simulink model "AIV_robot"  (R2024b)
settings: Solver=VariableStepAuto  StartTime=0.0  StopTime=35  RelTol=1e-2
InitFcn:
  | %% Position Error parameter
  | goal_x = 18.5;
  | goal_y = 16;
  | 
  | s0 = sqrt(goal_x^2 + goal_y^2);
  | isGoal_dist = 1.0;
  | 
  | %% Velocity parameter
  | VelScaler = 15;
  | 
  | 
  | %% get bus
  | BusActors = Simulink.Bus;
  | BusActors = getBusActors(BusActors);
  | BusActorsActors = Simulink.Bus;
  | BusActorsActors= getBusActorsActors(BusActorsActors);
  | 
  | %% get agent
  | load("agent.mat")
model workspace (MAT data in the model file):
  firstWarning = 1
  originalScenarioChecksum = '7C1E912B2141DACB6907C14F620C989B'
libraries: simulink x13, drivingscenarioandsensors x8, simulink_extras x1, autolibshared x1, rllib x1
(part 1 of 9)
settings Model: Creator=9  LastModifiedBy=aa007
settings SolverCC: DateTimeAtSimulationTimeZero=[]  ZeroCrossControl=EnableAll  ZeroCrossAlgorithm=Adaptive  MinimalZcImpactIntegration=on
settings DebuggingCC: ParameterOverflowMsg=warning  ParameterPrecisionLossMsg=none

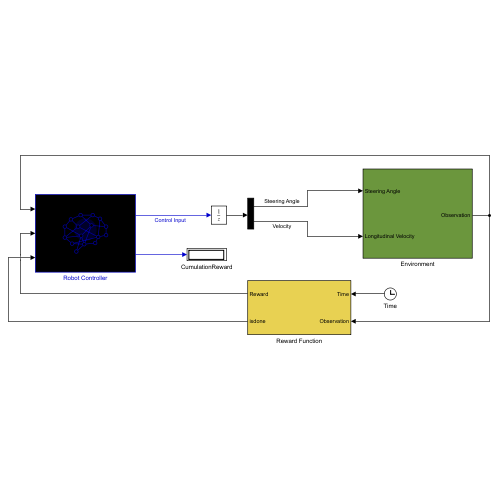
[thumbnail: Simulink's stored preview of the top-level diagram]
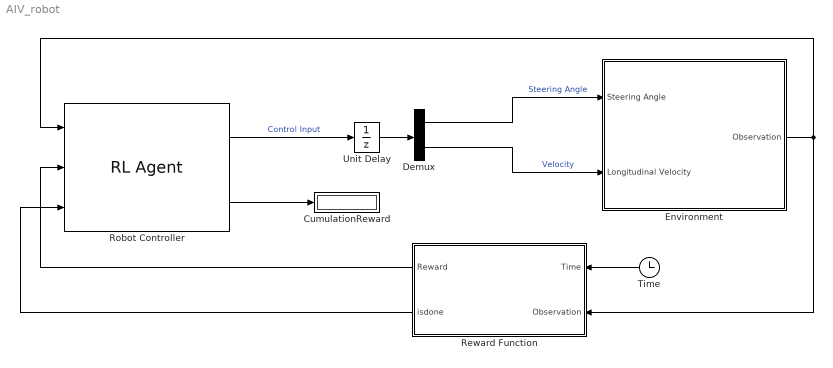
== system AIV_robot ==
  CumulationReward : Display
  Demux : Demux  Outputs=2
  Environment : Subsystem
  Reward Function : Subsystem
  Robot Controller : rllib/RL Agent  Agent=agent  ExternalActionAsInput=off  ProvideLastAction=off  ProvideCumRwd=on  TreatAsDirectFeedthrough=on  UseStrictObservationDataTypes=off
  Time : Clock
  Unit Delay : UnitDelay  SampleTime=-1  HasFrameUpgradeWarning=on
  wires:
  Reward Function/1(Reward) -> Robot Controller/2
  Demux/1 -> Environment/1(Steering Angle)  "Steering Angle"
  Demux/2 -> Environment/2(Longitudinal Velocity)  "Velocity"
  Time/1 -> Reward Function/1(Time)
  Environment/1(Observation) -> Reward Function/2(Observation), Robot Controller/1
  Reward Function/2(isdone) -> Robot Controller/3
  Robot Controller/2 -> CumulationReward/1
  Robot Controller/1 -> Unit Delay/1  "Control Input"
  Unit Delay/1 -> Demux/1

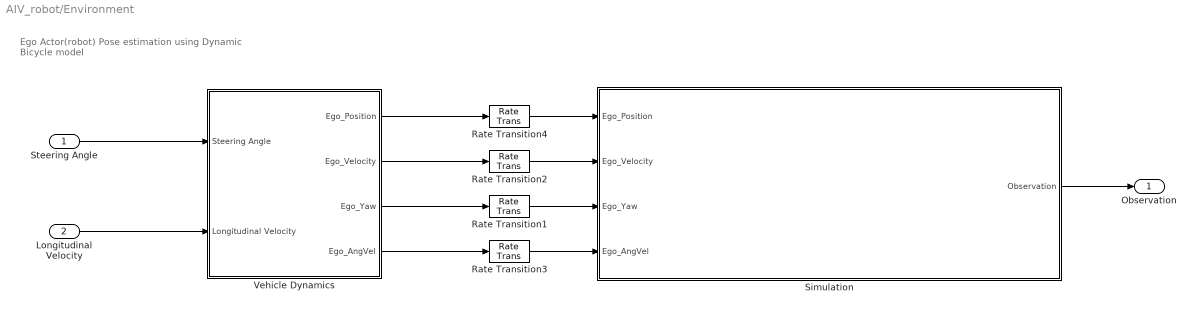
== system AIV_robot/Environment ==
  note: Ego Actor(robot) Pose estimation
      | using Dynamic Bicycle model
  Steering Angle : Inport
  Longitudinal Velocity : Inport  Port=2
  Rate Transition{1..4} (4 alike) : RateTransition
  Simulation : Subsystem
  Vehicle Dynamics : Subsystem
  Observation : Outport
  wires:
  Vehicle Dynamics/1(Ego_Position) -> Rate Transition4/1
  Vehicle Dynamics/2(Ego_Velocity) -> Rate Transition2/1
  Vehicle Dynamics/3(Ego_Yaw) -> Rate Transition1/1
  Vehicle Dynamics/4(Ego_AngVel) -> Rate Transition3/1
  Steering Angle/1 -> Vehicle Dynamics/1(Steering Angle)
  Longitudinal Velocity/1 -> Vehicle Dynamics/2(Longitudinal Velocity)
  Simulation/1(Observation) -> Observation/1
  Rate Transition2/1 -> Simulation/2(Ego_Velocity)
  Rate Transition1/1 -> Simulation/3(Ego_Yaw)
  Rate Transition3/1 -> Simulation/4(Ego_AngVel)
  Rate Transition4/1 -> Simulation/1(Ego_Position)

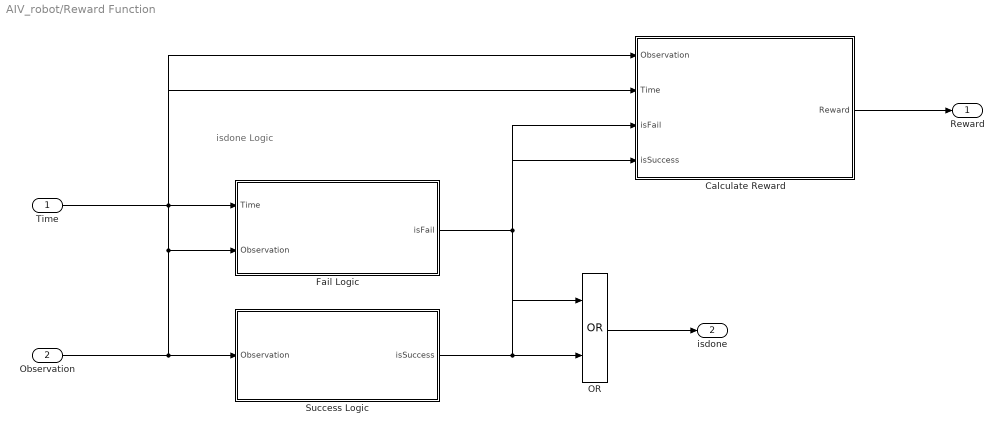
== system AIV_robot/Reward Function ==
  note: isdone Logic
  Time : Inport
  Observation : Inport  Port=2
  Calculate Reward : Subsystem
  Fail Logic : Subsystem
  OR : Logic  Operator=OR  AllPortsSameDT=off  OutDataTypeStr=boolean
  Success Logic : Subsystem
  Reward : Outport
  isdone : Outport  Port=2
  wires:
  Time/1 -> Fail Logic/1(Time), Calculate Reward/2(Time)
  Observation/1 -> Calculate Reward/1(Observation), Fail Logic/2(Observation), Success Logic/1(Observation)
  Fail Logic/1(isFail) -> OR/1, Calculate Reward/3(isFail)
  Success Logic/1(isSuccess) -> Calculate Reward/4(isSuccess), OR/2
  OR/1 -> isdone/1
  Calculate Reward/1(Reward) -> Reward/1

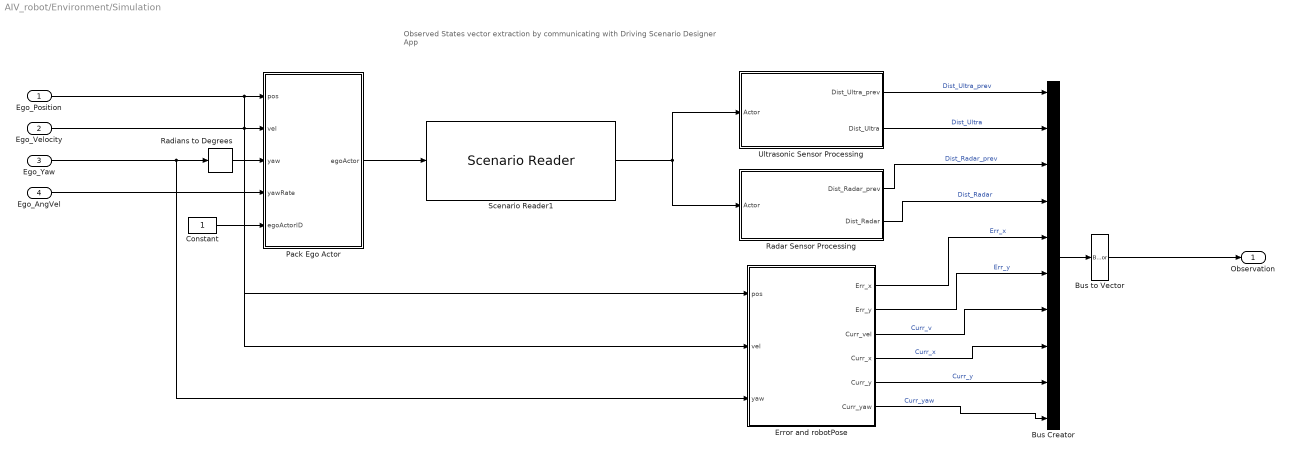
== system AIV_robot/Environment/Simulation ==
  note: Observed States vector extraction
      | by communicating with Driving Scenario Designer App
  Ego_Position : Inport
  Ego_Velocity : Inport  Port=2
  Ego_Yaw : Inport  Port=3
  Ego_AngVel : Inport  Port=4
  Bus Creator : BusCreator  Inputs=10
  Bus to Vector : BusToVector
  Constant : Constant
  Error and robotPose : Subsystem
  Pack Ego Actor : MATLAB Function  Priority=-1  TreatAsAtomicUnit=on
  Radar Sensor Processing : Subsystem
  Radians to Degrees : simulink_extras/Transformations/Radians to Degrees
  Scenario Reader1 : drivingscenarioandsensors/Scenario Reader  Priority=-1  ScenarioSource=From file  ScenarioFileName=C:\Users\aa007\OneDrive\바탕화~1-DESKTOP-L2TT5UE-65992184\ai_ws\ai_ws\scenario.mat  ScenarioVariableName=data  OutputCoordinateSystem=Vehicle coordinates  EgoVehicleSource=Input port  EgoVehicleActorID=1  OrientVehiclesOnRoad=on  OutputEgoVehiclePose=off  OutputEgoVehicleState=off  SampleTime=0.1  LaneBoundaryOutput=None  LaneBoundaryDistance=0:0.5:9.5  LaneBoundaryLocation=Center of lane markings  BusNameSource=Auto  BusName=BusActors  BusNumActorsSource=Scenario  BusNumActors=100  BusName2Source=Auto  BusName2=BusLaneBoundaries  BusNumLaneBoundariesSource=Scenario  BusNumLaneBoundaries=10  BusName3Source=Auto  BusName3=BusEgoActor  BusName4Source=Auto  BusName4=BusEgoState  ShowCoordinateLabels=on  SimulateUsing=Interpreted execution
  Ultrasonic Sensor Processing : Subsystem
  Observation : Outport
  wires:
  Ego_Position/1 -> Pack Ego Actor/1(pos), Error and robotPose/1(pos)
  Ego_Velocity/1 -> Error and robotPose/2(vel), Pack Ego Actor/2(vel)
  Ego_Yaw/1 -> Error and robotPose/3(yaw), Radians to Degrees/1
  Ego_AngVel/1 -> Pack Ego Actor/4(yawRate)
  Radians to Degrees/1 -> Pack Ego Actor/3(yaw)
  Ultrasonic Sensor Processing/1(Dist_Ultra_prev) -> Bus Creator/1  "Dist_Ultra_prev"
  Radar Sensor Processing/1(Dist_Radar_prev) -> Bus Creator/3  "Dist_Radar_prev"
  Bus Creator/1 -> Bus to Vector/1
  Ultrasonic Sensor Processing/2(Dist_Ultra) -> Bus Creator/2  "Dist_Ultra"
  Radar Sensor Processing/2(Dist_Radar) -> Bus Creator/4  "Dist_Radar"
  Error and robotPose/1(Err_x) -> Bus Creator/5  "Err_x"
  Error and robotPose/2(Err_y) -> Bus Creator/6  "Err_y"
  Constant/1 -> Pack Ego Actor/5(egoActorID)
  Pack Ego Actor/1(egoActor) -> Scenario Reader1/1
  Scenario Reader1/1 -> Ultrasonic Sensor Processing/1(Actor), Radar Sensor Processing/1(Actor)
  Bus to Vector/1 -> Observation/1
  Error and robotPose/3(Curr_vel) -> Bus Creator/7  "Curr_v"
  Error and robotPose/4(Curr_x) -> Bus Creator/8  "Curr_x"
  Error and robotPose/5(Curr_y) -> Bus Creator/9  "Curr_y"
  Error and robotPose/6(Curr_yaw) -> Bus Creator/10  "Curr_yaw"

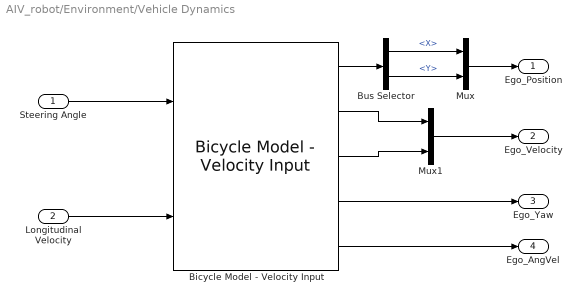
== system AIV_robot/Environment/Vehicle Dynamics ==
  Steering Angle : Inport
  Longitudinal Velocity : Inport  Port=2
  Bicycle Model - Velocity Input : autolibshared/Bicycle Model - Velocity Input  trackMode=Single (bicycle)  inputMode=External longitudinal velocity  frontSteerMode=on  rearSteerMode=off  windMode=off  muMode=off  extFMode=off  extMMode=off  aMode=3  NF=2  NR=2  m=150  a=0.22  b=0.22  h=0.35  X_o=0  xdot_o=0  CalphaMode=off  sigmaMode=on  w=[1.4,1.4]  Cy_f=8000  Cy_r=7500  sigma_f=.1  sigma_r=.1  alpha_f_brk=[-.1 .1]  Cy_f_data=[-9e3 9e3]  alpha_r_brk=[-.1 .1]  Cy_r_data=[-9e3 9e3]  Y_o=0  ydot_o=0  Izz=2000  psi_o=0  r_o=0  Af=2  Cd=.3  Cl=.1  Cpm=.1  beta_w=[0 0.01:0.01:0.3]  Cs=[0 0.01:0.01:0.3]  Cym=[0 1e-6:0.01:0.3]  Pabs=101325  Tair=273  g=9.81  mu=1  xdot_tol=.01  Fznom=5000  Fxtire_sat=1e6  Fytire_sat=1e6  longOff=0  latOff=0  vertOff=0
      settings: LibrarySourceBlock=drivingscenarioandsensors/Bicycle Model - Velocity Input
  Bus Selector : BusSelector  OutputSignals=InertFrm.FrntAxl.Disp.X,InertFrm.FrntAxl.Disp.Y
  Mux : Mux  Inputs=2
  Mux1 : Mux  Inputs=2
  Ego_Position : Outport
  Ego_Velocity : Outport  Port=2
  Ego_Yaw : Outport  Port=3
  Ego_AngVel : Outport  Port=4
  wires:
  Bicycle Model - Velocity Input/1 -> Bus Selector/1
  Bus Selector/1 -> Mux/1  "<X>"
  Bus Selector/2 -> Mux/2  "<Y>"
  Mux/1 -> Ego_Position/1
  Steering Angle/1 -> Bicycle Model - Velocity Input/1
  Longitudinal Velocity/1 -> Bicycle Model - Velocity Input/2
  Bicycle Model - Velocity Input/2 -> Mux1/1
  Bicycle Model - Velocity Input/3 -> Mux1/2
  Mux1/1 -> Ego_Velocity/1
  Bicycle Model - Velocity Input/4 -> Ego_Yaw/1
  Bicycle Model - Velocity Input/5 -> Ego_AngVel/1

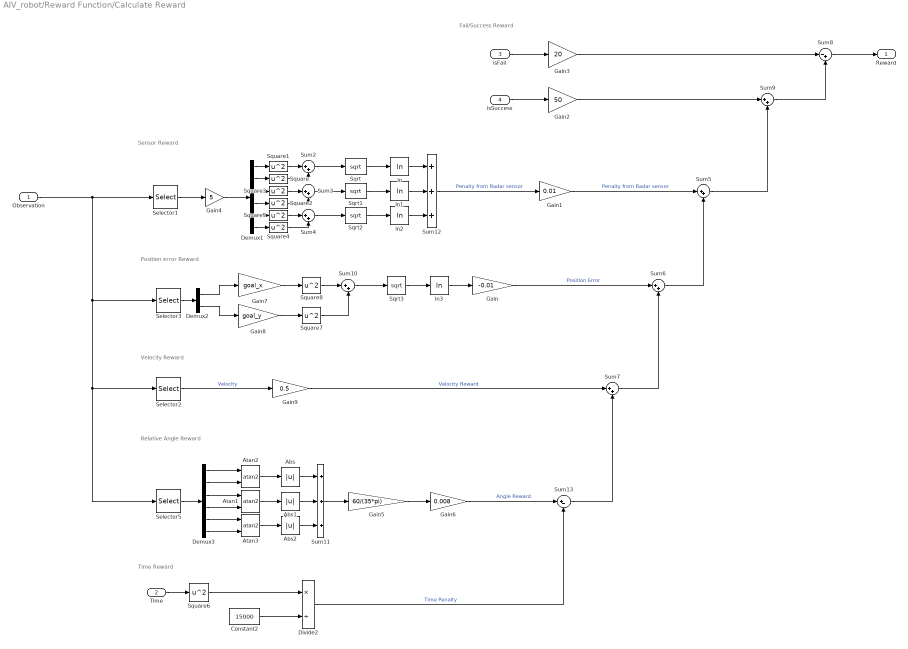
== system AIV_robot/Reward Function/Calculate Reward ==
  note: Sensor Reward
  note: Time Reward
  note: Fail/Success Reward
  note: Position error Reward
  note: Velocity Reward
  note: Relative Angle Reward
  Observation : Inport
  Time : Inport  Port=2
  isFail : Inport  Port=3
  isSuccess : Inport  Port=4
  Abs : Abs  SaturateOnIntegerOverflow=off
  Abs1 : Abs  SaturateOnIntegerOverflow=off
  Abs2 : Abs  SaturateOnIntegerOverflow=off
  Atan1 : Trigonometry  Operator=atan2
  Atan2 : Trigonometry  Operator=atan2
  Atan3 : Trigonometry  Operator=atan2
  Constant2 : Constant  Value=15000
  Demux1 : Demux  Outputs=6
  Demux2 : Demux  Outputs=2
  Demux3 : Demux  Outputs=6
  Divide2 : Product  Inputs=*/
  Gain : Gain  Gain=-0.01
  Gain1 : Gain  Gain=0.01
  Gain2 : Gain  Gain=50
  Gain3 : Gain  Gain=20
  Gain4 : Gain  Gain=5
  Gain5 : Gain  Gain=60/(35*pi)
  Gain6 : Gain  Gain=0.008
  Gain7 : Gain  Gain=goal_x
  Gain8 : Gain  Gain=goal_y
  Gain9 : Gain  Gain=0.5
  Selector1 : Selector  NumberOfDimensions=2  InputPortWidth=27  IndexOptions=Index vector (dialog),Index vector (dialog)  Indices=[23:28],1  OutputSizes=1,1
  Selector2 : Selector  NumberOfDimensions=2  InputPortWidth=27  IndexOptions=Index vector (dialog),Index vector (dialog)  Indices=35,1  OutputSizes=1,1
  Selector3 : Selector  NumberOfDimensions=2  InputPortWidth=27  IndexOptions=Index vector (dialog),Index vector (dialog)  Indices=[33 34],1  OutputSizes=1,1
  Selector5 : Selector  NumberOfDimensions=2  InputPortWidth=27  IndexOptions=Index vector (dialog),Index vector (dialog)  Indices=[23:28],1  OutputSizes=1,1
  Sqrt{,1..3} (4 alike) : Sqrt
  Square{,1..8} (9 alike) : Math  Operator=square
  Sum{2..7,9..10} (8 alike) : Sum  Inputs=|++
  Sum11 : Sum  Inputs=+++
  Sum12 : Sum  Inputs=+++
  Sum13 : Sum  Inputs=|+-
  Sum8 : Sum  Inputs=|-+
  ln{,1..3} (4 alike) : Math  Operator=log
  Reward : Outport
  wires:
  Observation/1 -> Selector1/1, Selector3/1, Selector5/1, Selector2/1
  Square/1 -> Sum2/2
  Square1/1 -> Sum2/1
  Sqrt/1 -> ln/1
  Sum4/1 -> Sqrt2/1
  Square5/1 -> Sum4/1
  Demux1/5 -> Square5/1
  Demux1/6 -> Square4/1
  Demux1/2 -> Square/1
  Demux1/4 -> Square2/1
  Sqrt2/1 -> ln2/1
  Selector1/1 -> Gain4/1
  Square4/1 -> Sum4/2
  Sqrt1/1 -> ln1/1
  Square3/1 -> Sum3/1
  Demux1/1 -> Square1/1
  Square2/1 -> Sum3/2
  Demux1/3 -> Square3/1
  Sum3/1 -> Sqrt1/1
  Sum2/1 -> Sqrt/1
  Sum12/1 -> Gain1/1  "Penalty from Radar sensor"
  Time/1 -> Square6/1
  Square6/1 -> Divide2/1
  Constant2/1 -> Divide2/2
  Gain1/1 -> Sum5/1  "Penalty from Radar sensor"
  isSuccess/1 -> Gain2/1
  isFail/1 -> Gain3/1
  Gain3/1 -> Sum8/1
  Gain2/1 -> Sum9/1
  Sum9/1 -> Sum8/2
  Sum8/1 -> Reward/1
  Sqrt3/1 -> ln3/1
  ln3/1 -> Gain/1
  Demux2/1 -> Gain7/1
  Square8/1 -> Sum10/1
  Selector3/1 -> Demux2/1
  Demux2/2 -> Gain8/1
  Sum10/1 -> Sqrt3/1
  Square7/1 -> Sum10/2
  ln/1 -> Sum12/1
  ln1/1 -> Sum12/2
  ln2/1 -> Sum12/3
  Sum5/1 -> Sum9/2
  Gain4/1 -> Demux1/1
  Selector2/1 -> Gain9/1  "Velocity"
  Selector5/1 -> Demux3/1
  Demux3/1 -> Atan2/1
  Demux3/2 -> Atan2/2
  Demux3/3 -> Atan1/1
  Demux3/4 -> Atan1/2
  Demux3/5 -> Atan3/1
  Demux3/6 -> Atan3/2
  Atan2/1 -> Abs/1
  Atan1/1 -> Abs1/1
  Atan3/1 -> Abs2/1
  Abs/1 -> Sum11/1
  Abs1/1 -> Sum11/2
  Abs2/1 -> Sum11/3
  Sum11/1 -> Gain5/1
  Gain5/1 -> Gain6/1
  Gain7/1 -> Square8/1
  Gain8/1 -> Square7/1
  Gain/1 -> Sum6/1  "Position Error"
  Gain9/1 -> Sum7/1  "Velocity Reward"
  Sum7/1 -> Sum6/2
  Sum6/1 -> Sum5/2
  Gain6/1 -> Sum13/1  "Angle Reward"
  Sum13/1 -> Sum7/2
  Divide2/1 -> Sum13/2  "Time Penalty"

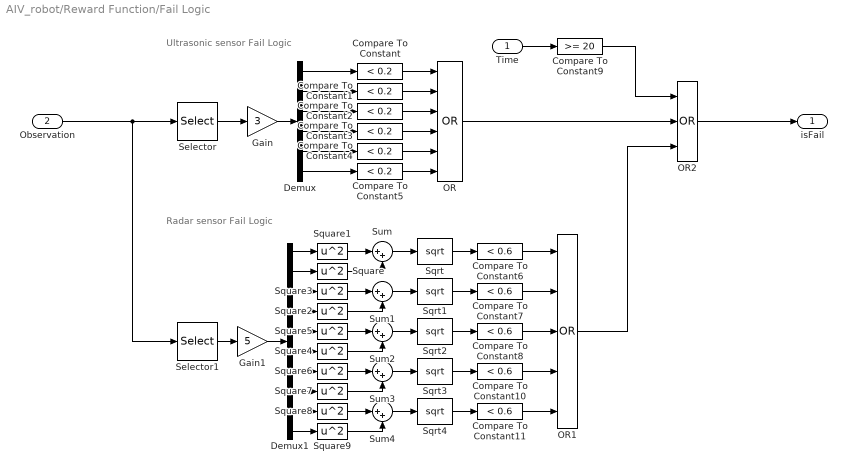
== system AIV_robot/Reward Function/Fail Logic ==
  note: Ultrasonic sensor Fail Logic
  note: Radar sensor Fail Logic
  Time : Inport
  Observation : Inport  Port=2
  Compare To Constant{,1..5} (6 alike) : simulink/Logic and Bit Operations/Compare To Constant  relop=<  const=0.2  OutDataTypeStr=boolean
  Compare To Constant{6..8,10..11} (5 alike) : simulink/Logic and Bit Operations/Compare To Constant  relop=<  const=0.6  OutDataTypeStr=boolean
  Compare To Constant9 : simulink/Logic and Bit Operations/Compare To Constant  relop=>=  const=20  OutDataTypeStr=boolean
  Demux : Demux  Outputs=6
  Demux1 : Demux  Outputs=10
  Gain : Gain  Gain=3
  Gain1 : Gain  Gain=5
  OR : Logic  Operator=OR  Inputs=6  AllPortsSameDT=off  OutDataTypeStr=boolean
  OR1 : Logic  Operator=OR  Inputs=5  AllPortsSameDT=off  OutDataTypeStr=boolean
  OR2 : Logic  Operator=OR  Inputs=3  AllPortsSameDT=off  OutDataTypeStr=boolean
  Selector : Selector  NumberOfDimensions=2  InputPortWidth=27  IndexOptions=Index vector (dialog),Index vector (dialog)  Indices=[7:12],1  OutputSizes=1,1
  Selector1 : Selector  NumberOfDimensions=2  InputPortWidth=27  IndexOptions=Index vector (dialog),Index vector (dialog)  Indices=[23:32],1  OutputSizes=1,1
  Sqrt{,1..4} (5 alike) : Sqrt
  Square{,1..9} (10 alike) : Math  Operator=square
  Sum{,1..4} (5 alike) : Sum  Inputs=|++
  isFail : Outport
  wires:
  Time/1 -> Compare To Constant9/1
  Observation/1 -> Selector1/1, Selector/1
  Selector/1 -> Gain/1
  Demux/1 -> Compare To Constant/1
  Demux/2 -> Compare To Constant1/1
  Demux/3 -> Compare To Constant2/1
  Demux/4 -> Compare To Constant3/1
  Demux/5 -> Compare To Constant4/1
  Demux/6 -> Compare To Constant5/1
  Compare To Constant5/1 -> OR/6
  Compare To Constant4/1 -> OR/5
  Compare To Constant3/1 -> OR/4
  Compare To Constant2/1 -> OR/3
  Compare To Constant1/1 -> OR/2
  Compare To Constant/1 -> OR/1
  OR/1 -> OR2/2
  Selector1/1 -> Gain1/1
  Sum/1 -> Sqrt/1
  Square/1 -> Sum/2
  Square1/1 -> Sum/1
  Demux1/1 -> Square1/1
  Demux1/2 -> Square/1
  Square3/1 -> Sum1/1
  Square2/1 -> Sum1/2
  Sum1/1 -> Sqrt1/1
  Demux1/3 -> Square3/1
  Demux1/4 -> Square2/1
  Demux1/6 -> Square4/1
  Square5/1 -> Sum2/1
  Square4/1 -> Sum2/2
  Demux1/5 -> Square5/1
  Sum2/1 -> Sqrt2/1
  Sqrt/1 -> Compare To Constant6/1
  Sqrt2/1 -> Compare To Constant8/1
  Sqrt1/1 -> Compare To Constant7/1
  Compare To Constant6/1 -> OR1/1
  Compare To Constant7/1 -> OR1/2
  Compare To Constant8/1 -> OR1/3
  Compare To Constant9/1 -> OR2/1
  OR2/1 -> isFail/1
  Demux1/7 -> Square6/1
  Demux1/8 -> Square7/1
  Demux1/9 -> Square8/1
  Demux1/10 -> Square9/1
  Sqrt3/1 -> Compare To Constant10/1
  Sqrt4/1 -> Compare To Constant11/1
  Sum4/1 -> Sqrt4/1
  Square9/1 -> Sum4/2
  Square8/1 -> Sum4/1
  Sum3/1 -> Sqrt3/1
  Square7/1 -> Sum3/2
  Square6/1 -> Sum3/1
  Compare To Constant10/1 -> OR1/4
  Compare To Constant11/1 -> OR1/5
  OR1/1 -> OR2/3
  Gain/1 -> Demux/1
  Gain1/1 -> Demux1/1

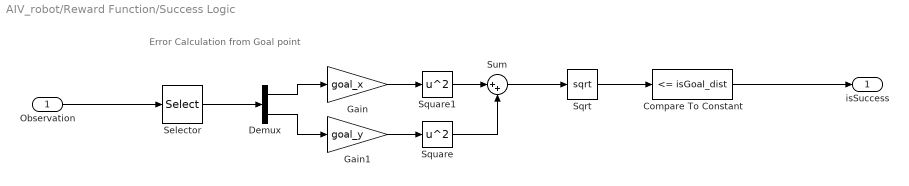
== system AIV_robot/Reward Function/Success Logic ==
  note: Error Calculation from Goal point
  Observation : Inport
  Compare To Constant : simulink/Logic and Bit Operations/Compare To Constant  relop=<=  const=isGoal_dist  OutDataTypeStr=boolean
  Demux : Demux  Outputs=2
  Gain : Gain  Gain=goal_x
  Gain1 : Gain  Gain=goal_y
  Selector : Selector  NumberOfDimensions=2  InputPortWidth=27  IndexOptions=Index vector (dialog),Index vector (dialog)  Indices=[33 34],1  OutputSizes=1,1
  Sqrt : Sqrt
  Square : Math  Operator=square
  Square1 : Math  Operator=square
  Sum : Sum  Inputs=|++
  isSuccess : Outport
  wires:
  Observation/1 -> Selector/1
  Selector/1 -> Demux/1
  Demux/2 -> Gain1/1
  Demux/1 -> Gain/1
  Square1/1 -> Sum/1
  Square/1 -> Sum/2
  Sum/1 -> Sqrt/1
  Sqrt/1 -> Compare To Constant/1
  Compare To Constant/1 -> isSuccess/1
  Gain/1 -> Square1/1
  Gain1/1 -> Square/1

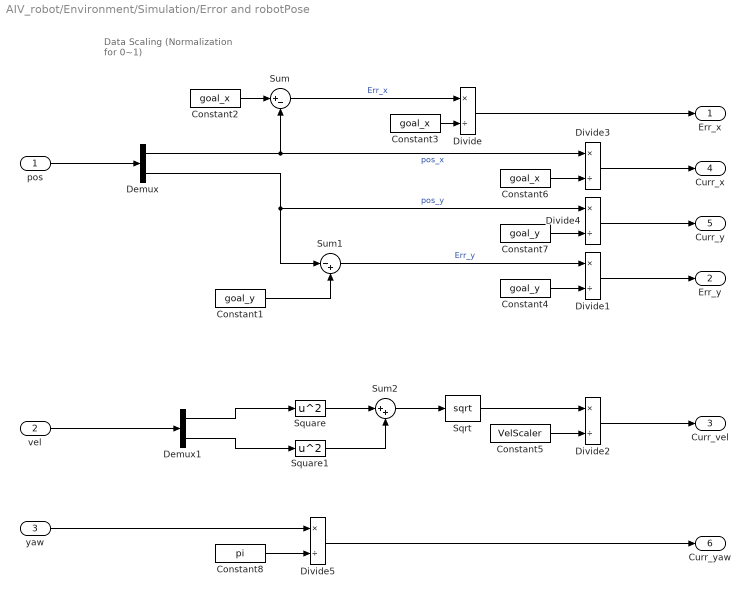
== system AIV_robot/Environment/Simulation/Error and robotPose ==
  note: Data Scaling
      | (Normalization for 0~1)
  pos : Inport
  vel : Inport  Port=2
  yaw : Inport  Port=3
  Constant1 : Constant  Value=goal_y
  Constant2 : Constant  Value=goal_x
  Constant3 : Constant  Value=goal_x
  Constant4 : Constant  Value=goal_y
  Constant5 : Constant  Value=VelScaler
  Constant6 : Constant  Value=goal_x
  Constant7 : Constant  Value=goal_y
  Constant8 : Constant  Value=pi
  Demux : Demux  Outputs=2
  Demux1 : Demux  Outputs=2
  Divide{,1..5} (6 alike) : Product  Inputs=*/
  Sqrt : Sqrt
  Square : Math  Operator=square
  Square1 : Math  Operator=square
  Sum : Sum  Inputs=|+-
  Sum1 : Sum  Inputs=|-+
  Sum2 : Sum  Inputs=|++
  Err_x : Outport
  Err_y : Outport  Port=2
  Curr_vel : Outport  Port=3
  Curr_x : Outport  Port=4
  Curr_y : Outport  Port=5
  Curr_yaw : Outport  Port=6
  wires:
  Sum2/1 -> Sqrt/1
  pos/1 -> Demux/1
  Demux1/1 -> Square/1
  Demux1/2 -> Square1/1
  Square1/1 -> Sum2/2
  Square/1 -> Sum2/1
  Sqrt/1 -> Divide2/1
  Sum/1 -> Divide/1  "Err_x"
  vel/1 -> Demux1/1
  Constant2/1 -> Sum/1
  Demux/1 -> Divide3/1, Sum/2  "pos_x"
  Demux/2 -> Sum1/1, Divide4/1  "pos_y"
  Constant1/1 -> Sum1/2
  Constant3/1 -> Divide/2
  Divide/1 -> Err_x/1
  Sum1/1 -> Divide1/1  "Err_y"
  Divide1/1 -> Err_y/1
  Constant4/1 -> Divide1/2
  Constant5/1 -> Divide2/2
  Divide2/1 -> Curr_vel/1
  Constant6/1 -> Divide3/2
  Constant7/1 -> Divide4/2
  Divide3/1 -> Curr_x/1
  Divide4/1 -> Curr_y/1
  yaw/1 -> Divide5/1
  Constant8/1 -> Divide5/2
  Divide5/1 -> Curr_yaw/1
